simulink model "lecture05d_planar_vehicle_model"  (R2024a)
settings: Solver=VariableStepAuto  StartTime=0.0  StopTime=t_final  MaxStep=deltaTMax  RelTol=1e-3
undefined symbols (not defined in the file or in its folder): GEOMETRY
libraries: PlanarVehicle x2
settings Model: Creator=Christopher  LastModifiedBy=chris
settings SolverCC: AlgebraicLoopSolver=TrustRegion
settings DataIOCC: ReturnWorkspaceOutputs=off
settings DebuggingCC: UnconnectedInputMsg=warning  UnconnectedOutputMsg=warning  UnconnectedLineMsg=warning  ArithmeticOperatorsInVariantConditions=warning
settings ModelReferenceCC: EnableRefExpFcnMdlSchedulingChecks=on
settings SFSimCC: CustomCodeUndefinedFunction=UseInterfaceOnly
settings RTWCC: GPUComputeCapability=3.5
settings SimscapeCC: EditingMode=Restricted

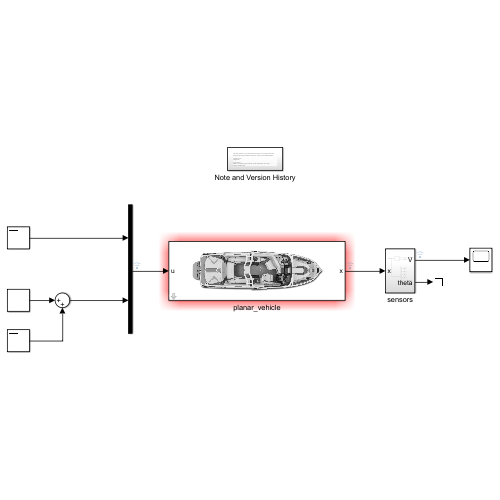
[thumbnail: Simulink's stored preview of the top-level diagram]
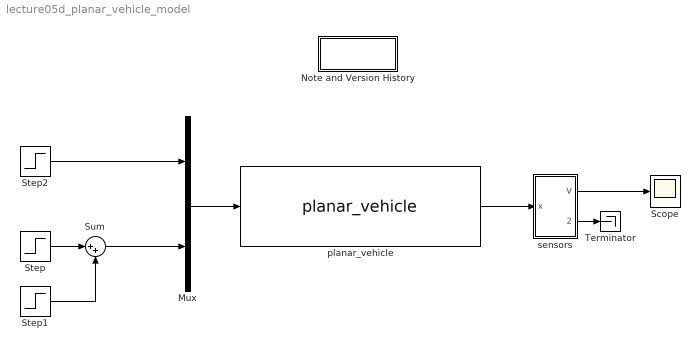
== system lecture05d_planar_vehicle_model ==
  Mux : Mux  Inputs=2
  Note and Version History : Subsystem
  Scope : Scope
  Step : Step  Time=10  SampleTime=0
  Step1 : Step  Time=30  After=-1  SampleTime=0
  Step2 : Step  Time=90  Before=1  After=0  SampleTime=0
  Sum : Sum  Inputs=|++
  Terminator : Terminator
  planar_vehicle : PlanarVehicle/planar_vehicle  m=GEOMETRY.mass  Ib=GEOMETRY.Ib  Fmax=PROPULSION.Fmax  Mmax=PROPULSION.Mmax  x0=SIMULATION.X_0  CT=ENVIRONMENT.CT  CR=ENVIRONMENT.CR
  sensors : Subsystem
  wires:
  planar_vehicle/1 -> sensors/1(x)
  Mux/1 -> planar_vehicle/1
  Step2/1 -> Mux/1
  Sum/1 -> Mux/2
  sensors/1(V) -> Scope/1
  Step/1 -> Sum/1
  Step1/1 -> Sum/2
  sensors/2(theta) -> Terminator/1

== system lecture05d_planar_vehicle_model/Note and Version History ==
  note: This has a dependency on the PlanarVehicle.slx library. See YouTube video entitled 'Obtaining and Using the MatlabLum Repository' at https://youtu.be/5ROS2-4ShmI .
      |
      | Christopher Lum
      | lum@uw.edu
      |
      | Version History
      | 03/28/21: Created from final_project/p2. Greatly simplified for lecture notes
      | 01/07/25: Updated notes.

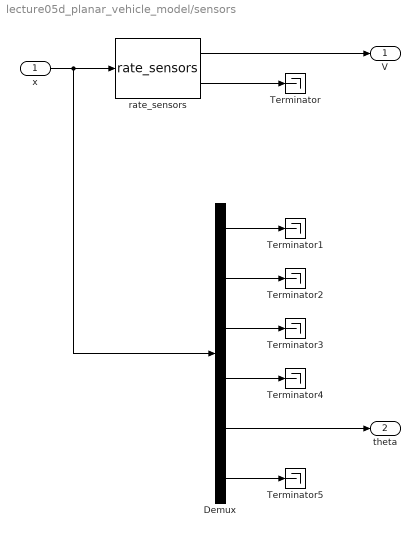
== system lecture05d_planar_vehicle_model/sensors ==
  x : Inport
  Demux : Demux  Outputs=6
  Terminator{,1..5} (6 alike) : Terminator
  rate_sensors : PlanarVehicle/rate_sensors
  V : Outport  VectorParamsAs1DForOutWhenUnconnected=off
  theta : Outport  Port=2  VectorParamsAs1DForOutWhenUnconnected=off
  wires:
  x/1 -> Demux/1, rate_sensors/1
  rate_sensors/1 -> V/1
  Demux/5 -> theta/1
  rate_sensors/2 -> Terminator/1
  Demux/1 -> Terminator1/1
  Demux/2 -> Terminator2/1
  Demux/3 -> Terminator3/1
  Demux/4 -> Terminator4/1
  Demux/6 -> Terminator5/1
